simulink model "TST_AccPed_DrvDemDes"  (R2016b)
settings: Solver=FixedStepDiscrete  StartTime=0.0  StopTime=simTime  FixedStep=sampleTime  RelTol=1e-3
values from neighbouring files (symbols this model uses):
  testCase = 1    [initTST_AccPed_DrvDemDes_001.m]    (also in initTST_AccPed_DrvDemDes_002.m = 2; initTST_AccPed_DrvDemDes_003.m = 3; initTST_AccPed_DrvDemDes_004.m = 4; initTST_AccPed_DrvDemDes_005.m = 5)
libraries: simulink x61, UnitTest_Lib x54
(part 2 of 2)

== system TST_AccPed_DrvDemDes/simulationInput/testSignals_R001 ==
  BC : BusCreator  Inputs=22
  spec_APP_r : FromWorkspace  VariableName=testSig_APP_r  Interpolate=off  OutputAfterFinalValue=Holding final value
  spec_AccPed_facCompAcs : FromWorkspace  VariableName=testSig_AccPed_facCompAcs  Interpolate=off  OutputAfterFinalValue=Holding final value
  spec_AccPed_rBrk50_mp : FromWorkspace  VariableName=testSig_AccPed_rBrk50_mp  Interpolate=off  OutputAfterFinalValue=Holding final value
  spec_AccPed_rTrq : FromWorkspace  VariableName=testSig_AccPed_rTrq  Interpolate=off  OutputAfterFinalValue=Holding final value
  spec_AccPed_stBrkDes : FromWorkspace  VariableName=testSig_AccPed_stBrkDes  Interpolate=off  OutputAfterFinalValue=Holding final value
  spec_AccPed_stBrkDes_mp : FromWorkspace  VariableName=testSig_AccPed_stBrkDes_mp  Interpolate=off  OutputAfterFinalValue=Holding final value
  spec_AccPed_stMS : FromWorkspace  VariableName=testSig_AccPed_stMS  Interpolate=off  OutputAfterFinalValue=Holding final value
  spec_AccPed_trqComp : FromWorkspace  VariableName=testSig_AccPed_trqComp  Interpolate=off  OutputAfterFinalValue=Holding final value
  spec_AccPed_trqDesAct : FromWorkspace  VariableName=testSig_AccPed_trqDesAct  Interpolate=off  OutputAfterFinalValue=Holding final value
  spec_AccPed_trqDesPull : FromWorkspace  VariableName=testSig_AccPed_trqDesPull  Interpolate=off  OutputAfterFinalValue=Holding final value
  spec_AccPed_trqDifBrk_mp : FromWorkspace  VariableName=testSig_AccPed_trqDifBrk_mp  Interpolate=off  OutputAfterFinalValue=Holding final value
  spec_AccPed_trqLimMax : FromWorkspace  VariableName=testSig_AccPed_trqLimMax  Interpolate=off  OutputAfterFinalValue=Holding final value
  spec_Brk_st : FromWorkspace  VariableName=testSig_Brk_st  Interpolate=off  OutputAfterFinalValue=Holding final value
  spec_CoME_trqDesComp : FromWorkspace  VariableName=testSig_CoME_trqDesComp  Interpolate=off  OutputAfterFinalValue=Holding final value
  spec_DrvDem_swtDrvNGovActv : FromWorkspace  VariableName=testSig_DrvDem_swtDrvNGovActv  Interpolate=off  OutputAfterFinalValue=Holding final value
  spec_EBrk_st : FromWorkspace  VariableName=testSig_EBrk_st  Interpolate=off  OutputAfterFinalValue=Holding final value
  spec_Epm_nEng : FromWorkspace  VariableName=testSig_Epm_nEng  Interpolate=off  OutputAfterFinalValue=Holding final value
  spec_GlbDa_vX : FromWorkspace  VariableName=testSig_GlbDa_vX  Interpolate=off  OutputAfterFinalValue=Holding final value
  spec_PT_stTraRevGear : FromWorkspace  VariableName=testSig_PT_stTraRevGear  Interpolate=off  OutputAfterFinalValue=Holding final value
  spec_PT_trqWhlMinEng : FromWorkspace  VariableName=testSig_PT_trqWhlMinEng  Interpolate=off  OutputAfterFinalValue=Holding final value
  spec_PT_trqWhlMinEngBrk : FromWorkspace  VariableName=testSig_PT_trqWhlMinEngBrk  Interpolate=off  OutputAfterFinalValue=Holding final value
  spec_VehMot_stPrpAccPed : FromWorkspace  VariableName=testSig_VehMot_stPrpAccPed  Interpolate=off  OutputAfterFinalValue=Holding final value
  testSignals : Outport
  wires:
  BC/1 -> testSignals/1
  spec_PT_trqWhlMinEng/1 -> BC/1  "testSig_PT_trqWhlMinEng"
  spec_APP_r/1 -> BC/2  "testSig_APP_r"
  spec_Epm_nEng/1 -> BC/3  "testSig_Epm_nEng"
  spec_GlbDa_vX/1 -> BC/4  "testSig_GlbDa_vX"
  spec_CoME_trqDesComp/1 -> BC/5  "testSig_CoME_trqDesComp"
  spec_DrvDem_swtDrvNGovActv/1 -> BC/6  "testSig_DrvDem_swtDrvNGovActv"
  spec_Brk_st/1 -> BC/7  "testSig_Brk_st"
  spec_EBrk_st/1 -> BC/8  "testSig_EBrk_st"
  spec_PT_trqWhlMinEngBrk/1 -> BC/9  "testSig_PT_trqWhlMinEngBrk"
  spec_AccPed_trqLimMax/1 -> BC/10  "testSig_AccPed_trqLimMax"
  spec_AccPed_rTrq/1 -> BC/11  "testSig_AccPed_rTrq"
  spec_AccPed_stMS/1 -> BC/12  "testSig_AccPed_stMS"
  spec_PT_stTraRevGear/1 -> BC/13  "testSig_PT_stTraRevGear"
  spec_AccPed_trqDesAct/1 -> BC/14  "testSig_AccPed_trqDesAct"
  spec_VehMot_stPrpAccPed/1 -> BC/15  "testSig_VehMot_stPrpAccPed"
  spec_AccPed_facCompAcs/1 -> BC/16  "testSig_AccPed_facCompAcs"
  spec_AccPed_trqComp/1 -> BC/17  "testSig_AccPed_trqComp"
  spec_AccPed_stBrkDes/1 -> BC/18  "testSig_AccPed_stBrkDes"
  spec_AccPed_stBrkDes_mp/1 -> BC/19  "testSig_AccPed_stBrkDes_mp"
  spec_AccPed_trqDifBrk_mp/1 -> BC/20  "testSig_AccPed_trqDifBrk_mp"
  spec_AccPed_rBrk50_mp/1 -> BC/21  "testSig_AccPed_rBrk50_mp"
  spec_AccPed_trqDesPull/1 -> BC/22  "testSig_AccPed_trqDesPull"

== system TST_AccPed_DrvDemDes/simulationInput/testSignals_R002 ==
  BC : BusCreator  Inputs=22
  spec_APP_r : FromWorkspace  VariableName=testSig_APP_r  Interpolate=off  OutputAfterFinalValue=Holding final value
  spec_AccPed_facCompAcs : FromWorkspace  VariableName=testSig_AccPed_facCompAcs  Interpolate=off  OutputAfterFinalValue=Holding final value
  spec_AccPed_rBrk50_mp : FromWorkspace  VariableName=testSig_AccPed_rBrk50_mp  Interpolate=off  OutputAfterFinalValue=Holding final value
  spec_AccPed_rTrq : FromWorkspace  VariableName=testSig_AccPed_rTrq  Interpolate=off  OutputAfterFinalValue=Holding final value
  spec_AccPed_stBrkDes : FromWorkspace  VariableName=testSig_AccPed_stBrkDes  Interpolate=off  OutputAfterFinalValue=Holding final value
  spec_AccPed_stBrkDes_mp : FromWorkspace  VariableName=testSig_AccPed_stBrkDes_mp  Interpolate=off  OutputAfterFinalValue=Holding final value
  spec_AccPed_stMS : FromWorkspace  VariableName=testSig_AccPed_stMS  Interpolate=off  OutputAfterFinalValue=Holding final value
  spec_AccPed_trqComp : FromWorkspace  VariableName=testSig_AccPed_trqComp  Interpolate=off  OutputAfterFinalValue=Holding final value
  spec_AccPed_trqDesAct : FromWorkspace  VariableName=testSig_AccPed_trqDesAct  Interpolate=off  OutputAfterFinalValue=Holding final value
  spec_AccPed_trqDesPull : FromWorkspace  VariableName=testSig_AccPed_trqDesPull  Interpolate=off  OutputAfterFinalValue=Holding final value
  spec_AccPed_trqDifBrk_mp : FromWorkspace  VariableName=testSig_AccPed_trqDifBrk_mp  Interpolate=off  OutputAfterFinalValue=Holding final value
  spec_AccPed_trqLimMax : FromWorkspace  VariableName=testSig_AccPed_trqLimMax  Interpolate=off  OutputAfterFinalValue=Holding final value
  spec_Brk_st : FromWorkspace  VariableName=testSig_Brk_st  Interpolate=off  OutputAfterFinalValue=Holding final value
  spec_CoME_trqDesComp : FromWorkspace  VariableName=testSig_CoME_trqDesComp  Interpolate=off  OutputAfterFinalValue=Holding final value
  spec_DrvDem_swtDrvNGovActv : FromWorkspace  VariableName=testSig_DrvDem_swtDrvNGovActv  Interpolate=off  OutputAfterFinalValue=Holding final value
  spec_EBrk_st : FromWorkspace  VariableName=testSig_EBrk_st  Interpolate=off  OutputAfterFinalValue=Holding final value
  spec_Epm_nEng : FromWorkspace  VariableName=testSig_Epm_nEng  Interpolate=off  OutputAfterFinalValue=Holding final value
  spec_GlbDa_vX : FromWorkspace  VariableName=testSig_GlbDa_vX  Interpolate=off  OutputAfterFinalValue=Holding final value
  spec_PT_stTraRevGear : FromWorkspace  VariableName=testSig_PT_stTraRevGear  Interpolate=off  OutputAfterFinalValue=Holding final value
  spec_PT_trqWhlMinEng : FromWorkspace  VariableName=testSig_PT_trqWhlMinEng  Interpolate=off  OutputAfterFinalValue=Holding final value
  spec_PT_trqWhlMinEngBrk : FromWorkspace  VariableName=testSig_PT_trqWhlMinEngBrk  Interpolate=off  OutputAfterFinalValue=Holding final value
  spec_VehMot_stPrpAccPed : FromWorkspace  VariableName=testSig_VehMot_stPrpAccPed  Interpolate=off  OutputAfterFinalValue=Holding final value
  testSignals : Outport
  wires:
  BC/1 -> testSignals/1
  spec_PT_trqWhlMinEng/1 -> BC/1  "testSig_PT_trqWhlMinEng"
  spec_APP_r/1 -> BC/2  "testSig_APP_r"
  spec_Epm_nEng/1 -> BC/3  "testSig_Epm_nEng"
  spec_GlbDa_vX/1 -> BC/4  "testSig_GlbDa_vX"
  spec_CoME_trqDesComp/1 -> BC/5  "testSig_CoME_trqDesComp"
  spec_DrvDem_swtDrvNGovActv/1 -> BC/6  "testSig_DrvDem_swtDrvNGovActv"
  spec_Brk_st/1 -> BC/7  "testSig_Brk_st"
  spec_EBrk_st/1 -> BC/8  "testSig_EBrk_st"
  spec_PT_trqWhlMinEngBrk/1 -> BC/9  "testSig_PT_trqWhlMinEngBrk"
  spec_AccPed_trqLimMax/1 -> BC/10  "testSig_AccPed_trqLimMax"
  spec_AccPed_rTrq/1 -> BC/11  "testSig_AccPed_rTrq"
  spec_AccPed_stMS/1 -> BC/12  "testSig_AccPed_stMS"
  spec_PT_stTraRevGear/1 -> BC/13  "testSig_PT_stTraRevGear"
  spec_AccPed_trqDesAct/1 -> BC/14  "testSig_AccPed_trqDesAct"
  spec_VehMot_stPrpAccPed/1 -> BC/15  "testSig_VehMot_stPrpAccPed"
  spec_AccPed_facCompAcs/1 -> BC/16  "testSig_AccPed_facCompAcs"
  spec_AccPed_trqComp/1 -> BC/17  "testSig_AccPed_trqComp"
  spec_AccPed_stBrkDes/1 -> BC/18  "testSig_AccPed_stBrkDes"
  spec_AccPed_stBrkDes_mp/1 -> BC/19  "testSig_AccPed_stBrkDes_mp"
  spec_AccPed_trqDifBrk_mp/1 -> BC/20  "testSig_AccPed_trqDifBrk_mp"
  spec_AccPed_rBrk50_mp/1 -> BC/21  "testSig_AccPed_rBrk50_mp"
  spec_AccPed_trqDesPull/1 -> BC/22  "testSig_AccPed_trqDesPull"

== system TST_AccPed_DrvDemDes/simulationInput/testSignals_R003 ==
  BC : BusCreator  Inputs=22
  spec_APP_r : FromWorkspace  VariableName=testSig_APP_r  Interpolate=off  OutputAfterFinalValue=Holding final value
  spec_AccPed_facCompAcs : FromWorkspace  VariableName=testSig_AccPed_facCompAcs  Interpolate=off  OutputAfterFinalValue=Holding final value
  spec_AccPed_rBrk50_mp : FromWorkspace  VariableName=testSig_AccPed_rBrk50_mp  Interpolate=off  OutputAfterFinalValue=Holding final value
  spec_AccPed_rTrq : FromWorkspace  VariableName=testSig_AccPed_rTrq  Interpolate=off  OutputAfterFinalValue=Holding final value
  spec_AccPed_stBrkDes : FromWorkspace  VariableName=testSig_AccPed_stBrkDes  Interpolate=off  OutputAfterFinalValue=Holding final value
  spec_AccPed_stBrkDes_mp : FromWorkspace  VariableName=testSig_AccPed_stBrkDes_mp  Interpolate=off  OutputAfterFinalValue=Holding final value
  spec_AccPed_stMS : FromWorkspace  VariableName=testSig_AccPed_stMS  Interpolate=off  OutputAfterFinalValue=Holding final value
  spec_AccPed_trqComp : FromWorkspace  VariableName=testSig_AccPed_trqComp  Interpolate=off  OutputAfterFinalValue=Holding final value
  spec_AccPed_trqDesAct : FromWorkspace  VariableName=testSig_AccPed_trqDesAct  Interpolate=off  OutputAfterFinalValue=Holding final value
  spec_AccPed_trqDesPull : FromWorkspace  VariableName=testSig_AccPed_trqDesPull  Interpolate=off  OutputAfterFinalValue=Holding final value
  spec_AccPed_trqDifBrk_mp : FromWorkspace  VariableName=testSig_AccPed_trqDifBrk_mp  Interpolate=off  OutputAfterFinalValue=Holding final value
  spec_AccPed_trqLimMax : FromWorkspace  VariableName=testSig_AccPed_trqLimMax  Interpolate=off  OutputAfterFinalValue=Holding final value
  spec_Brk_st : FromWorkspace  VariableName=testSig_Brk_st  Interpolate=off  OutputAfterFinalValue=Holding final value
  spec_CoME_trqDesComp : FromWorkspace  VariableName=testSig_CoME_trqDesComp  Interpolate=off  OutputAfterFinalValue=Holding final value
  spec_DrvDem_swtDrvNGovActv : FromWorkspace  VariableName=testSig_DrvDem_swtDrvNGovActv  Interpolate=off  OutputAfterFinalValue=Holding final value
  spec_EBrk_st : FromWorkspace  VariableName=testSig_EBrk_st  Interpolate=off  OutputAfterFinalValue=Holding final value
  spec_Epm_nEng : FromWorkspace  VariableName=testSig_Epm_nEng  Interpolate=off  OutputAfterFinalValue=Holding final value
  spec_GlbDa_vX : FromWorkspace  VariableName=testSig_GlbDa_vX  Interpolate=off  OutputAfterFinalValue=Holding final value
  spec_PT_stTraRevGear : FromWorkspace  VariableName=testSig_PT_stTraRevGear  Interpolate=off  OutputAfterFinalValue=Holding final value
  spec_PT_trqWhlMinEng : FromWorkspace  VariableName=testSig_PT_trqWhlMinEng  Interpolate=off  OutputAfterFinalValue=Holding final value
  spec_PT_trqWhlMinEngBrk : FromWorkspace  VariableName=testSig_PT_trqWhlMinEngBrk  Interpolate=off  OutputAfterFinalValue=Holding final value
  spec_VehMot_stPrpAccPed : FromWorkspace  VariableName=testSig_VehMot_stPrpAccPed  Interpolate=off  OutputAfterFinalValue=Holding final value
  testSignals : Outport
  wires:
  BC/1 -> testSignals/1
  spec_PT_trqWhlMinEng/1 -> BC/1  "testSig_PT_trqWhlMinEng"
  spec_APP_r/1 -> BC/2  "testSig_APP_r"
  spec_Epm_nEng/1 -> BC/3  "testSig_Epm_nEng"
  spec_GlbDa_vX/1 -> BC/4  "testSig_GlbDa_vX"
  spec_CoME_trqDesComp/1 -> BC/5  "testSig_CoME_trqDesComp"
  spec_DrvDem_swtDrvNGovActv/1 -> BC/6  "testSig_DrvDem_swtDrvNGovActv"
  spec_Brk_st/1 -> BC/7  "testSig_Brk_st"
  spec_EBrk_st/1 -> BC/8  "testSig_EBrk_st"
  spec_PT_trqWhlMinEngBrk/1 -> BC/9  "testSig_PT_trqWhlMinEngBrk"
  spec_AccPed_trqLimMax/1 -> BC/10  "testSig_AccPed_trqLimMax"
  spec_AccPed_rTrq/1 -> BC/11  "testSig_AccPed_rTrq"
  spec_AccPed_stMS/1 -> BC/12  "testSig_AccPed_stMS"
  spec_PT_stTraRevGear/1 -> BC/13  "testSig_PT_stTraRevGear"
  spec_AccPed_trqDesAct/1 -> BC/14  "testSig_AccPed_trqDesAct"
  spec_VehMot_stPrpAccPed/1 -> BC/15  "testSig_VehMot_stPrpAccPed"
  spec_AccPed_facCompAcs/1 -> BC/16  "testSig_AccPed_facCompAcs"
  spec_AccPed_trqComp/1 -> BC/17  "testSig_AccPed_trqComp"
  spec_AccPed_stBrkDes/1 -> BC/18  "testSig_AccPed_stBrkDes"
  spec_AccPed_stBrkDes_mp/1 -> BC/19  "testSig_AccPed_stBrkDes_mp"
  spec_AccPed_trqDifBrk_mp/1 -> BC/20  "testSig_AccPed_trqDifBrk_mp"
  spec_AccPed_rBrk50_mp/1 -> BC/21  "testSig_AccPed_rBrk50_mp"
  spec_AccPed_trqDesPull/1 -> BC/22  "testSig_AccPed_trqDesPull"

== system TST_AccPed_DrvDemDes/simulationInput/testSignals_R004 ==
  BC : BusCreator  Inputs=22
  spec_APP_r : FromWorkspace  VariableName=testSig_APP_r  Interpolate=off  OutputAfterFinalValue=Holding final value
  spec_AccPed_facCompAcs : FromWorkspace  VariableName=testSig_AccPed_facCompAcs  Interpolate=off  OutputAfterFinalValue=Holding final value
  spec_AccPed_rBrk50_mp : FromWorkspace  VariableName=testSig_AccPed_rBrk50_mp  Interpolate=off  OutputAfterFinalValue=Holding final value
  spec_AccPed_rTrq : FromWorkspace  VariableName=testSig_AccPed_rTrq  Interpolate=off  OutputAfterFinalValue=Holding final value
  spec_AccPed_stBrkDes : FromWorkspace  VariableName=testSig_AccPed_stBrkDes  Interpolate=off  OutputAfterFinalValue=Holding final value
  spec_AccPed_stBrkDes_mp : FromWorkspace  VariableName=testSig_AccPed_stBrkDes_mp  Interpolate=off  OutputAfterFinalValue=Holding final value
  spec_AccPed_stMS : FromWorkspace  VariableName=testSig_AccPed_stMS  Interpolate=off  OutputAfterFinalValue=Holding final value
  spec_AccPed_trqComp : FromWorkspace  VariableName=testSig_AccPed_trqComp  Interpolate=off  OutputAfterFinalValue=Holding final value
  spec_AccPed_trqDesAct : FromWorkspace  VariableName=testSig_AccPed_trqDesAct  Interpolate=off  OutputAfterFinalValue=Holding final value
  spec_AccPed_trqDesPull : FromWorkspace  VariableName=testSig_AccPed_trqDesPull  Interpolate=off  OutputAfterFinalValue=Holding final value
  spec_AccPed_trqDifBrk_mp : FromWorkspace  VariableName=testSig_AccPed_trqDifBrk_mp  Interpolate=off  OutputAfterFinalValue=Holding final value
  spec_AccPed_trqLimMax : FromWorkspace  VariableName=testSig_AccPed_trqLimMax  Interpolate=off  OutputAfterFinalValue=Holding final value
  spec_Brk_st : FromWorkspace  VariableName=testSig_Brk_st  Interpolate=off  OutputAfterFinalValue=Holding final value
  spec_CoME_trqDesComp : FromWorkspace  VariableName=testSig_CoME_trqDesComp  Interpolate=off  OutputAfterFinalValue=Holding final value
  spec_DrvDem_swtDrvNGovActv : FromWorkspace  VariableName=testSig_DrvDem_swtDrvNGovActv  Interpolate=off  OutputAfterFinalValue=Holding final value
  spec_EBrk_st : FromWorkspace  VariableName=testSig_EBrk_st  Interpolate=off  OutputAfterFinalValue=Holding final value
  spec_Epm_nEng : FromWorkspace  VariableName=testSig_Epm_nEng  Interpolate=off  OutputAfterFinalValue=Holding final value
  spec_GlbDa_vX : FromWorkspace  VariableName=testSig_GlbDa_vX  Interpolate=off  OutputAfterFinalValue=Holding final value
  spec_PT_stTraRevGear : FromWorkspace  VariableName=testSig_PT_stTraRevGear  Interpolate=off  OutputAfterFinalValue=Holding final value
  spec_PT_trqWhlMinEng : FromWorkspace  VariableName=testSig_PT_trqWhlMinEng  Interpolate=off  OutputAfterFinalValue=Holding final value
  spec_PT_trqWhlMinEngBrk : FromWorkspace  VariableName=testSig_PT_trqWhlMinEngBrk  Interpolate=off  OutputAfterFinalValue=Holding final value
  spec_VehMot_stPrpAccPed : FromWorkspace  VariableName=testSig_VehMot_stPrpAccPed  Interpolate=off  OutputAfterFinalValue=Holding final value
  testSignals : Outport
  wires:
  BC/1 -> testSignals/1
  spec_PT_trqWhlMinEng/1 -> BC/1  "testSig_PT_trqWhlMinEng"
  spec_APP_r/1 -> BC/2  "testSig_APP_r"
  spec_Epm_nEng/1 -> BC/3  "testSig_Epm_nEng"
  spec_GlbDa_vX/1 -> BC/4  "testSig_GlbDa_vX"
  spec_CoME_trqDesComp/1 -> BC/5  "testSig_CoME_trqDesComp"
  spec_DrvDem_swtDrvNGovActv/1 -> BC/6  "testSig_DrvDem_swtDrvNGovActv"
  spec_Brk_st/1 -> BC/7  "testSig_Brk_st"
  spec_EBrk_st/1 -> BC/8  "testSig_EBrk_st"
  spec_PT_trqWhlMinEngBrk/1 -> BC/9  "testSig_PT_trqWhlMinEngBrk"
  spec_AccPed_trqLimMax/1 -> BC/10  "testSig_AccPed_trqLimMax"
  spec_AccPed_rTrq/1 -> BC/11  "testSig_AccPed_rTrq"
  spec_AccPed_stMS/1 -> BC/12  "testSig_AccPed_stMS"
  spec_PT_stTraRevGear/1 -> BC/13  "testSig_PT_stTraRevGear"
  spec_AccPed_trqDesAct/1 -> BC/14  "testSig_AccPed_trqDesAct"
  spec_VehMot_stPrpAccPed/1 -> BC/15  "testSig_VehMot_stPrpAccPed"
  spec_AccPed_facCompAcs/1 -> BC/16  "testSig_AccPed_facCompAcs"
  spec_AccPed_trqComp/1 -> BC/17  "testSig_AccPed_trqComp"
  spec_AccPed_stBrkDes/1 -> BC/18  "testSig_AccPed_stBrkDes"
  spec_AccPed_stBrkDes_mp/1 -> BC/19  "testSig_AccPed_stBrkDes_mp"
  spec_AccPed_trqDifBrk_mp/1 -> BC/20  "testSig_AccPed_trqDifBrk_mp"
  spec_AccPed_rBrk50_mp/1 -> BC/21  "testSig_AccPed_rBrk50_mp"
  spec_AccPed_trqDesPull/1 -> BC/22  "testSig_AccPed_trqDesPull"

== system TST_AccPed_DrvDemDes/simulationInput/testSignals_R005 ==
  BC : BusCreator  Inputs=22
  spec_APP_r : FromWorkspace  VariableName=testSig_APP_r  Interpolate=off  OutputAfterFinalValue=Holding final value
  spec_AccPed_facCompAcs : FromWorkspace  VariableName=testSig_AccPed_facCompAcs  Interpolate=off  OutputAfterFinalValue=Holding final value
  spec_AccPed_rBrk50_mp : FromWorkspace  VariableName=testSig_AccPed_rBrk50_mp  Interpolate=off  OutputAfterFinalValue=Holding final value
  spec_AccPed_rTrq : FromWorkspace  VariableName=testSig_AccPed_rTrq  Interpolate=off  OutputAfterFinalValue=Holding final value
  spec_AccPed_stBrkDes : FromWorkspace  VariableName=testSig_AccPed_stBrkDes  Interpolate=off  OutputAfterFinalValue=Holding final value
  spec_AccPed_stBrkDes_mp : FromWorkspace  VariableName=testSig_AccPed_stBrkDes_mp  Interpolate=off  OutputAfterFinalValue=Holding final value
  spec_AccPed_stMS : FromWorkspace  VariableName=testSig_AccPed_stMS  Interpolate=off  OutputAfterFinalValue=Holding final value
  spec_AccPed_trqComp : FromWorkspace  VariableName=testSig_AccPed_trqComp  Interpolate=off  OutputAfterFinalValue=Holding final value
  spec_AccPed_trqDesAct : FromWorkspace  VariableName=testSig_AccPed_trqDesAct  Interpolate=off  OutputAfterFinalValue=Holding final value
  spec_AccPed_trqDesPull : FromWorkspace  VariableName=testSig_AccPed_trqDesPull  Interpolate=off  OutputAfterFinalValue=Holding final value
  spec_AccPed_trqDifBrk_mp : FromWorkspace  VariableName=testSig_AccPed_trqDifBrk_mp  Interpolate=off  OutputAfterFinalValue=Holding final value
  spec_AccPed_trqLimMax : FromWorkspace  VariableName=testSig_AccPed_trqLimMax  Interpolate=off  OutputAfterFinalValue=Holding final value
  spec_Brk_st : FromWorkspace  VariableName=testSig_Brk_st  Interpolate=off  OutputAfterFinalValue=Holding final value
  spec_CoME_trqDesComp : FromWorkspace  VariableName=testSig_CoME_trqDesComp  Interpolate=off  OutputAfterFinalValue=Holding final value
  spec_DrvDem_swtDrvNGovActv : FromWorkspace  VariableName=testSig_DrvDem_swtDrvNGovActv  Interpolate=off  OutputAfterFinalValue=Holding final value
  spec_EBrk_st : FromWorkspace  VariableName=testSig_EBrk_st  Interpolate=off  OutputAfterFinalValue=Holding final value
  spec_Epm_nEng : FromWorkspace  VariableName=testSig_Epm_nEng  Interpolate=off  OutputAfterFinalValue=Holding final value
  spec_GlbDa_vX : FromWorkspace  VariableName=testSig_GlbDa_vX  Interpolate=off  OutputAfterFinalValue=Holding final value
  spec_PT_stTraRevGear : FromWorkspace  VariableName=testSig_PT_stTraRevGear  Interpolate=off  OutputAfterFinalValue=Holding final value
  spec_PT_trqWhlMinEng : FromWorkspace  VariableName=testSig_PT_trqWhlMinEng  Interpolate=off  OutputAfterFinalValue=Holding final value
  spec_PT_trqWhlMinEngBrk : FromWorkspace  VariableName=testSig_PT_trqWhlMinEngBrk  Interpolate=off  OutputAfterFinalValue=Holding final value
  spec_VehMot_stPrpAccPed : FromWorkspace  VariableName=testSig_VehMot_stPrpAccPed  Interpolate=off  OutputAfterFinalValue=Holding final value
  testSignals : Outport
  wires:
  BC/1 -> testSignals/1
  spec_PT_trqWhlMinEng/1 -> BC/1  "testSig_PT_trqWhlMinEng"
  spec_APP_r/1 -> BC/2  "testSig_APP_r"
  spec_Epm_nEng/1 -> BC/3  "testSig_Epm_nEng"
  spec_GlbDa_vX/1 -> BC/4  "testSig_GlbDa_vX"
  spec_CoME_trqDesComp/1 -> BC/5  "testSig_CoME_trqDesComp"
  spec_DrvDem_swtDrvNGovActv/1 -> BC/6  "testSig_DrvDem_swtDrvNGovActv"
  spec_Brk_st/1 -> BC/7  "testSig_Brk_st"
  spec_EBrk_st/1 -> BC/8  "testSig_EBrk_st"
  spec_PT_trqWhlMinEngBrk/1 -> BC/9  "testSig_PT_trqWhlMinEngBrk"
  spec_AccPed_trqLimMax/1 -> BC/10  "testSig_AccPed_trqLimMax"
  spec_AccPed_rTrq/1 -> BC/11  "testSig_AccPed_rTrq"
  spec_AccPed_stMS/1 -> BC/12  "testSig_AccPed_stMS"
  spec_PT_stTraRevGear/1 -> BC/13  "testSig_PT_stTraRevGear"
  spec_AccPed_trqDesAct/1 -> BC/14  "testSig_AccPed_trqDesAct"
  spec_VehMot_stPrpAccPed/1 -> BC/15  "testSig_VehMot_stPrpAccPed"
  spec_AccPed_facCompAcs/1 -> BC/16  "testSig_AccPed_facCompAcs"
  spec_AccPed_trqComp/1 -> BC/17  "testSig_AccPed_trqComp"
  spec_AccPed_stBrkDes/1 -> BC/18  "testSig_AccPed_stBrkDes"
  spec_AccPed_stBrkDes_mp/1 -> BC/19  "testSig_AccPed_stBrkDes_mp"
  spec_AccPed_trqDifBrk_mp/1 -> BC/20  "testSig_AccPed_trqDifBrk_mp"
  spec_AccPed_rBrk50_mp/1 -> BC/21  "testSig_AccPed_rBrk50_mp"
  spec_AccPed_trqDesPull/1 -> BC/22  "testSig_AccPed_trqDesPull"

== system TST_AccPed_DrvDemDes/simulationInput/testSignals_R006 ==
  BC : BusCreator  Inputs=22
  spec_APP_r : FromWorkspace  VariableName=testSig_APP_r  Interpolate=off  OutputAfterFinalValue=Holding final value
  spec_AccPed_facCompAcs : FromWorkspace  VariableName=testSig_AccPed_facCompAcs  Interpolate=off  OutputAfterFinalValue=Holding final value
  spec_AccPed_rBrk50_mp : FromWorkspace  VariableName=testSig_AccPed_rBrk50_mp  Interpolate=off  OutputAfterFinalValue=Holding final value
  spec_AccPed_rTrq : FromWorkspace  VariableName=testSig_AccPed_rTrq  Interpolate=off  OutputAfterFinalValue=Holding final value
  spec_AccPed_stBrkDes : FromWorkspace  VariableName=testSig_AccPed_stBrkDes  Interpolate=off  OutputAfterFinalValue=Holding final value
  spec_AccPed_stBrkDes_mp : FromWorkspace  VariableName=testSig_AccPed_stBrkDes_mp  Interpolate=off  OutputAfterFinalValue=Holding final value
  spec_AccPed_stMS : FromWorkspace  VariableName=testSig_AccPed_stMS  Interpolate=off  OutputAfterFinalValue=Holding final value
  spec_AccPed_trqComp : FromWorkspace  VariableName=testSig_AccPed_trqComp  Interpolate=off  OutputAfterFinalValue=Holding final value
  spec_AccPed_trqDesAct : FromWorkspace  VariableName=testSig_AccPed_trqDesAct  Interpolate=off  OutputAfterFinalValue=Holding final value
  spec_AccPed_trqDesPull : FromWorkspace  VariableName=testSig_AccPed_trqDesPull  Interpolate=off  OutputAfterFinalValue=Holding final value
  spec_AccPed_trqDifBrk_mp : FromWorkspace  VariableName=testSig_AccPed_trqDifBrk_mp  Interpolate=off  OutputAfterFinalValue=Holding final value
  spec_AccPed_trqLimMax : FromWorkspace  VariableName=testSig_AccPed_trqLimMax  Interpolate=off  OutputAfterFinalValue=Holding final value
  spec_Brk_st : FromWorkspace  VariableName=testSig_Brk_st  Interpolate=off  OutputAfterFinalValue=Holding final value
  spec_CoME_trqDesComp : FromWorkspace  VariableName=testSig_CoME_trqDesComp  Interpolate=off  OutputAfterFinalValue=Holding final value
  spec_DrvDem_swtDrvNGovActv : FromWorkspace  VariableName=testSig_DrvDem_swtDrvNGovActv  Interpolate=off  OutputAfterFinalValue=Holding final value
  spec_EBrk_st : FromWorkspace  VariableName=testSig_EBrk_st  Interpolate=off  OutputAfterFinalValue=Holding final value
  spec_Epm_nEng : FromWorkspace  VariableName=testSig_Epm_nEng  Interpolate=off  OutputAfterFinalValue=Holding final value
  spec_GlbDa_vX : FromWorkspace  VariableName=testSig_GlbDa_vX  Interpolate=off  OutputAfterFinalValue=Holding final value
  spec_PT_stTraRevGear : FromWorkspace  VariableName=testSig_PT_stTraRevGear  Interpolate=off  OutputAfterFinalValue=Holding final value
  spec_PT_trqWhlMinEng : FromWorkspace  VariableName=testSig_PT_trqWhlMinEng  Interpolate=off  OutputAfterFinalValue=Holding final value
  spec_PT_trqWhlMinEngBrk : FromWorkspace  VariableName=testSig_PT_trqWhlMinEngBrk  Interpolate=off  OutputAfterFinalValue=Holding final value
  spec_VehMot_stPrpAccPed : FromWorkspace  VariableName=testSig_VehMot_stPrpAccPed  Interpolate=off  OutputAfterFinalValue=Holding final value
  testSignals : Outport
  wires:
  BC/1 -> testSignals/1
  spec_PT_trqWhlMinEng/1 -> BC/1  "testSig_PT_trqWhlMinEng"
  spec_APP_r/1 -> BC/2  "testSig_APP_r"
  spec_Epm_nEng/1 -> BC/3  "testSig_Epm_nEng"
  spec_GlbDa_vX/1 -> BC/4  "testSig_GlbDa_vX"
  spec_CoME_trqDesComp/1 -> BC/5  "testSig_CoME_trqDesComp"
  spec_DrvDem_swtDrvNGovActv/1 -> BC/6  "testSig_DrvDem_swtDrvNGovActv"
  spec_Brk_st/1 -> BC/7  "testSig_Brk_st"
  spec_EBrk_st/1 -> BC/8  "testSig_EBrk_st"
  spec_PT_trqWhlMinEngBrk/1 -> BC/9  "testSig_PT_trqWhlMinEngBrk"
  spec_AccPed_trqLimMax/1 -> BC/10  "testSig_AccPed_trqLimMax"
  spec_AccPed_rTrq/1 -> BC/11  "testSig_AccPed_rTrq"
  spec_AccPed_stMS/1 -> BC/12  "testSig_AccPed_stMS"
  spec_PT_stTraRevGear/1 -> BC/13  "testSig_PT_stTraRevGear"
  spec_AccPed_trqDesAct/1 -> BC/14  "testSig_AccPed_trqDesAct"
  spec_VehMot_stPrpAccPed/1 -> BC/15  "testSig_VehMot_stPrpAccPed"
  spec_AccPed_facCompAcs/1 -> BC/16  "testSig_AccPed_facCompAcs"
  spec_AccPed_trqComp/1 -> BC/17  "testSig_AccPed_trqComp"
  spec_AccPed_stBrkDes/1 -> BC/18  "testSig_AccPed_stBrkDes"
  spec_AccPed_stBrkDes_mp/1 -> BC/19  "testSig_AccPed_stBrkDes_mp"
  spec_AccPed_trqDifBrk_mp/1 -> BC/20  "testSig_AccPed_trqDifBrk_mp"
  spec_AccPed_rBrk50_mp/1 -> BC/21  "testSig_AccPed_rBrk50_mp"
  spec_AccPed_trqDesPull/1 -> BC/22  "testSig_AccPed_trqDesPull"

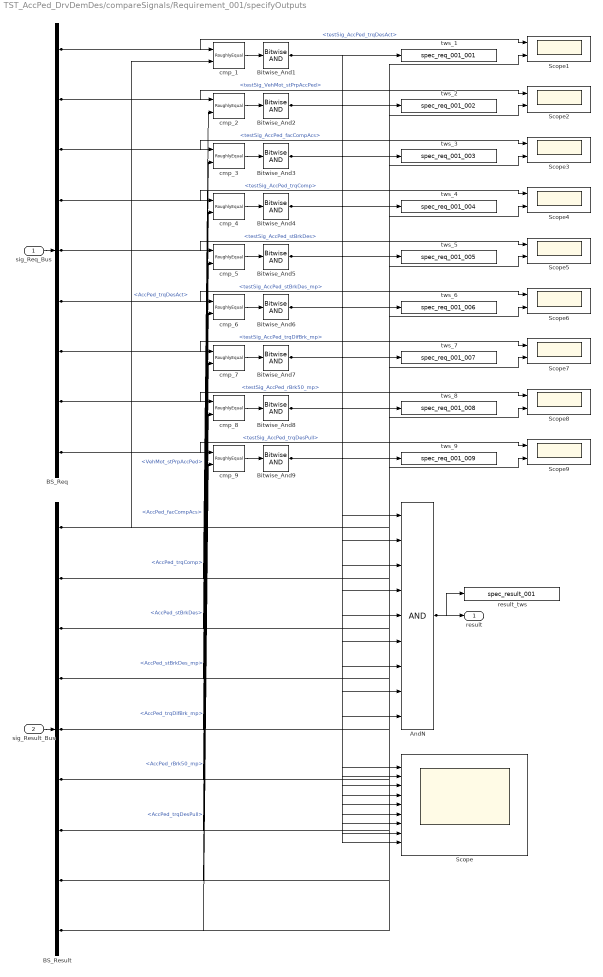
== system TST_AccPed_DrvDemDes/compareSignals/Requirement_001/specifyOutputs ==
  sig_Req_Bus : Inport
  sig_Result_Bus : Inport  Port=2
  AndN : Logic  Inputs=9
  BS_Req : BusSelector  OutputSignals=testSig_AccPed_trqDesAct,testSig_VehMot_stPrpAccPed,testSig_AccPed_facCompAcs,testSig_AccPed_trqComp,testSig_AccPed_stBrkDes,testSig_AccPed_stBrkDes_mp,testSig_AccPed_trqDifBrk_mp,testSig_AccPed_rBrk50_mp,testSig_AccPed_trqDesPull
  BS_Result : BusSelector  OutputSignals=AccPed_trqDesAct,VehMot_stPrpAccPed,AccPed_facCompAcs,AccPed_trqComp,AccPed_stBrkDes,AccPed_stBrkDes_mp,AccPed_trqDifBrk_mp,AccPed_rBrk50_mp,AccPed_trqDesPull
  Bitwise_And{1..9} (9 alike) : simulink/Logic and Bit Operations/Bitwise Operator  logicop=AND  UseBitMask=off  BitMask=bin2dec('11011001')  BitMaskRealWorld=Stored Integer
  Scope : Scope  NumInputPorts=9
  Scope{1..9} (9 alike) : Scope  NumInputPorts=2
  cmp_{1..9} (9 alike) : UnitTest_Lib/RoughlyEqual  slope=0.1
  result_tws : ToWorkspace  VariableName=spec_result_001
  tws_1 : ToWorkspace  VariableName=spec_req_001_001
  tws_2 : ToWorkspace  VariableName=spec_req_001_002
  tws_3 : ToWorkspace  VariableName=spec_req_001_003
  tws_4 : ToWorkspace  VariableName=spec_req_001_004
  tws_5 : ToWorkspace  VariableName=spec_req_001_005
  tws_6 : ToWorkspace  VariableName=spec_req_001_006
  tws_7 : ToWorkspace  VariableName=spec_req_001_007
  tws_8 : ToWorkspace  VariableName=spec_req_001_008
  tws_9 : ToWorkspace  VariableName=spec_req_001_009
  result : Outport
  wires:
  sig_Req_Bus/1 -> BS_Req/1
  sig_Result_Bus/1 -> BS_Result/1
  AndN/1 -> result/1, result_tws/1
  BS_Req/1 -> cmp_1/1, Scope1/1  "<testSig_AccPed_trqDesAct>"
  BS_Result/1 -> cmp_1/2, Scope1/2  "<AccPed_trqDesAct>"
  cmp_1/1 -> Bitwise_And1/1
  Bitwise_And1/1 -> tws_1/1, AndN/1, Scope/1
  BS_Req/2 -> cmp_2/1, Scope2/1  "<testSig_VehMot_stPrpAccPed>"
  BS_Result/2 -> cmp_2/2, Scope2/2  "<VehMot_stPrpAccPed>"
  cmp_2/1 -> Bitwise_And2/1
  Bitwise_And2/1 -> tws_2/1, AndN/2, Scope/2
  BS_Req/3 -> cmp_3/1, Scope3/1  "<testSig_AccPed_facCompAcs>"
  BS_Result/3 -> cmp_3/2, Scope3/2  "<AccPed_facCompAcs>"
  cmp_3/1 -> Bitwise_And3/1
  Bitwise_And3/1 -> tws_3/1, AndN/3, Scope/3
  BS_Req/4 -> cmp_4/1, Scope4/1  "<testSig_AccPed_trqComp>"
  BS_Result/4 -> cmp_4/2, Scope4/2  "<AccPed_trqComp>"
  cmp_4/1 -> Bitwise_And4/1
  Bitwise_And4/1 -> tws_4/1, AndN/4, Scope/4
  BS_Req/5 -> cmp_5/1, Scope5/1  "<testSig_AccPed_stBrkDes>"
  BS_Result/5 -> cmp_5/2, Scope5/2  "<AccPed_stBrkDes>"
  cmp_5/1 -> Bitwise_And5/1
  Bitwise_And5/1 -> tws_5/1, AndN/5, Scope/5
  BS_Req/6 -> cmp_6/1, Scope6/1  "<testSig_AccPed_stBrkDes_mp>"
  BS_Result/6 -> cmp_6/2, Scope6/2  "<AccPed_stBrkDes_mp>"
  cmp_6/1 -> Bitwise_And6/1
  Bitwise_And6/1 -> tws_6/1, AndN/6, Scope/6
  BS_Req/7 -> cmp_7/1, Scope7/1  "<testSig_AccPed_trqDifBrk_mp>"
  BS_Result/7 -> cmp_7/2, Scope7/2  "<AccPed_trqDifBrk_mp>"
  cmp_7/1 -> Bitwise_And7/1
  Bitwise_And7/1 -> tws_7/1, AndN/7, Scope/7
  BS_Req/8 -> cmp_8/1, Scope8/1  "<testSig_AccPed_rBrk50_mp>"
  BS_Result/8 -> cmp_8/2, Scope8/2  "<AccPed_rBrk50_mp>"
  cmp_8/1 -> Bitwise_And8/1
  Bitwise_And8/1 -> tws_8/1, AndN/8, Scope/8
  BS_Req/9 -> cmp_9/1, Scope9/1  "<testSig_AccPed_trqDesPull>"
  BS_Result/9 -> cmp_9/2, Scope9/2  "<AccPed_trqDesPull>"
  cmp_9/1 -> Bitwise_And9/1
  Bitwise_And9/1 -> tws_9/1, AndN/9, Scope/9

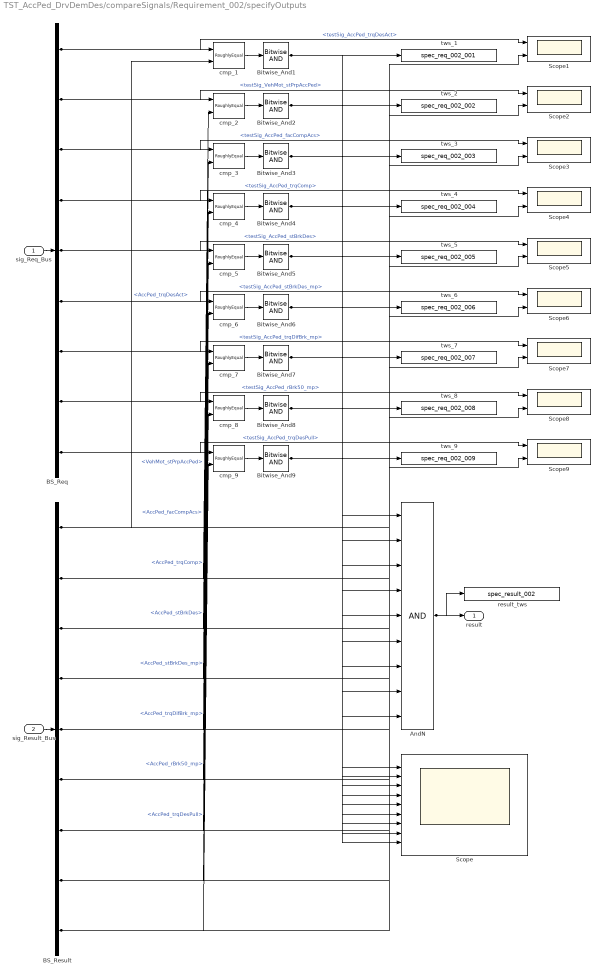
== system TST_AccPed_DrvDemDes/compareSignals/Requirement_002/specifyOutputs ==
  sig_Req_Bus : Inport
  sig_Result_Bus : Inport  Port=2
  AndN : Logic  Inputs=9
  BS_Req : BusSelector  OutputSignals=testSig_AccPed_trqDesAct,testSig_VehMot_stPrpAccPed,testSig_AccPed_facCompAcs,testSig_AccPed_trqComp,testSig_AccPed_stBrkDes,testSig_AccPed_stBrkDes_mp,testSig_AccPed_trqDifBrk_mp,testSig_AccPed_rBrk50_mp,testSig_AccPed_trqDesPull
  BS_Result : BusSelector  OutputSignals=AccPed_trqDesAct,VehMot_stPrpAccPed,AccPed_facCompAcs,AccPed_trqComp,AccPed_stBrkDes,AccPed_stBrkDes_mp,AccPed_trqDifBrk_mp,AccPed_rBrk50_mp,AccPed_trqDesPull
  Bitwise_And{1..9} (9 alike) : simulink/Logic and Bit Operations/Bitwise Operator  logicop=AND  UseBitMask=off  BitMask=bin2dec('11011001')  BitMaskRealWorld=Stored Integer
  Scope : Scope  NumInputPorts=9
  Scope{1..9} (9 alike) : Scope  NumInputPorts=2
  cmp_{1..9} (9 alike) : UnitTest_Lib/RoughlyEqual  slope=0.1
  result_tws : ToWorkspace  VariableName=spec_result_002
  tws_1 : ToWorkspace  VariableName=spec_req_002_001
  tws_2 : ToWorkspace  VariableName=spec_req_002_002
  tws_3 : ToWorkspace  VariableName=spec_req_002_003
  tws_4 : ToWorkspace  VariableName=spec_req_002_004
  tws_5 : ToWorkspace  VariableName=spec_req_002_005
  tws_6 : ToWorkspace  VariableName=spec_req_002_006
  tws_7 : ToWorkspace  VariableName=spec_req_002_007
  tws_8 : ToWorkspace  VariableName=spec_req_002_008
  tws_9 : ToWorkspace  VariableName=spec_req_002_009
  result : Outport
  wires:
  sig_Req_Bus/1 -> BS_Req/1
  sig_Result_Bus/1 -> BS_Result/1
  AndN/1 -> result/1, result_tws/1
  BS_Req/1 -> cmp_1/1, Scope1/1  "<testSig_AccPed_trqDesAct>"
  BS_Result/1 -> cmp_1/2, Scope1/2  "<AccPed_trqDesAct>"
  cmp_1/1 -> Bitwise_And1/1
  Bitwise_And1/1 -> tws_1/1, AndN/1, Scope/1
  BS_Req/2 -> cmp_2/1, Scope2/1  "<testSig_VehMot_stPrpAccPed>"
  BS_Result/2 -> cmp_2/2, Scope2/2  "<VehMot_stPrpAccPed>"
  cmp_2/1 -> Bitwise_And2/1
  Bitwise_And2/1 -> tws_2/1, AndN/2, Scope/2
  BS_Req/3 -> cmp_3/1, Scope3/1  "<testSig_AccPed_facCompAcs>"
  BS_Result/3 -> cmp_3/2, Scope3/2  "<AccPed_facCompAcs>"
  cmp_3/1 -> Bitwise_And3/1
  Bitwise_And3/1 -> tws_3/1, AndN/3, Scope/3
  BS_Req/4 -> cmp_4/1, Scope4/1  "<testSig_AccPed_trqComp>"
  BS_Result/4 -> cmp_4/2, Scope4/2  "<AccPed_trqComp>"
  cmp_4/1 -> Bitwise_And4/1
  Bitwise_And4/1 -> tws_4/1, AndN/4, Scope/4
  BS_Req/5 -> cmp_5/1, Scope5/1  "<testSig_AccPed_stBrkDes>"
  BS_Result/5 -> cmp_5/2, Scope5/2  "<AccPed_stBrkDes>"
  cmp_5/1 -> Bitwise_And5/1
  Bitwise_And5/1 -> tws_5/1, AndN/5, Scope/5
  BS_Req/6 -> cmp_6/1, Scope6/1  "<testSig_AccPed_stBrkDes_mp>"
  BS_Result/6 -> cmp_6/2, Scope6/2  "<AccPed_stBrkDes_mp>"
  cmp_6/1 -> Bitwise_And6/1
  Bitwise_And6/1 -> tws_6/1, AndN/6, Scope/6
  BS_Req/7 -> cmp_7/1, Scope7/1  "<testSig_AccPed_trqDifBrk_mp>"
  BS_Result/7 -> cmp_7/2, Scope7/2  "<AccPed_trqDifBrk_mp>"
  cmp_7/1 -> Bitwise_And7/1
  Bitwise_And7/1 -> tws_7/1, AndN/7, Scope/7
  BS_Req/8 -> cmp_8/1, Scope8/1  "<testSig_AccPed_rBrk50_mp>"
  BS_Result/8 -> cmp_8/2, Scope8/2  "<AccPed_rBrk50_mp>"
  cmp_8/1 -> Bitwise_And8/1
  Bitwise_And8/1 -> tws_8/1, AndN/8, Scope/8
  BS_Req/9 -> cmp_9/1, Scope9/1  "<testSig_AccPed_trqDesPull>"
  BS_Result/9 -> cmp_9/2, Scope9/2  "<AccPed_trqDesPull>"
  cmp_9/1 -> Bitwise_And9/1
  Bitwise_And9/1 -> tws_9/1, AndN/9, Scope/9

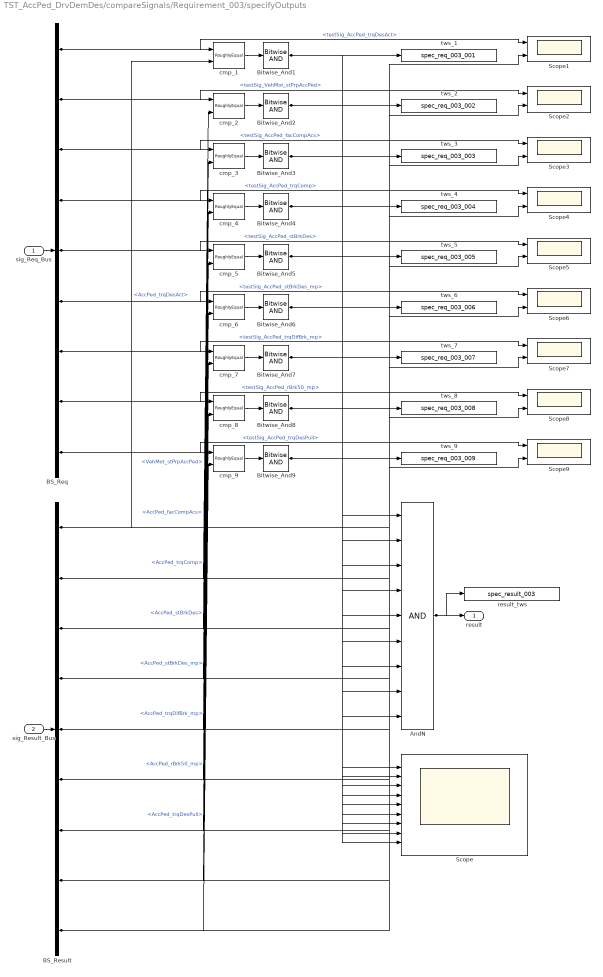
== system TST_AccPed_DrvDemDes/compareSignals/Requirement_003/specifyOutputs ==
  sig_Req_Bus : Inport
  sig_Result_Bus : Inport  Port=2
  AndN : Logic  Inputs=9
  BS_Req : BusSelector  OutputSignals=testSig_AccPed_trqDesAct,testSig_VehMot_stPrpAccPed,testSig_AccPed_facCompAcs,testSig_AccPed_trqComp,testSig_AccPed_stBrkDes,testSig_AccPed_stBrkDes_mp,testSig_AccPed_trqDifBrk_mp,testSig_AccPed_rBrk50_mp,testSig_AccPed_trqDesPull
  BS_Result : BusSelector  OutputSignals=AccPed_trqDesAct,VehMot_stPrpAccPed,AccPed_facCompAcs,AccPed_trqComp,AccPed_stBrkDes,AccPed_stBrkDes_mp,AccPed_trqDifBrk_mp,AccPed_rBrk50_mp,AccPed_trqDesPull
  Bitwise_And{1..9} (9 alike) : simulink/Logic and Bit Operations/Bitwise Operator  logicop=AND  UseBitMask=off  BitMask=bin2dec('11011001')  BitMaskRealWorld=Stored Integer
  Scope : Scope  NumInputPorts=9
  Scope{1..9} (9 alike) : Scope  NumInputPorts=2
  cmp_{1..9} (9 alike) : UnitTest_Lib/RoughlyEqual  slope=0.1
  result_tws : ToWorkspace  VariableName=spec_result_003
  tws_1 : ToWorkspace  VariableName=spec_req_003_001
  tws_2 : ToWorkspace  VariableName=spec_req_003_002
  tws_3 : ToWorkspace  VariableName=spec_req_003_003
  tws_4 : ToWorkspace  VariableName=spec_req_003_004
  tws_5 : ToWorkspace  VariableName=spec_req_003_005
  tws_6 : ToWorkspace  VariableName=spec_req_003_006
  tws_7 : ToWorkspace  VariableName=spec_req_003_007
  tws_8 : ToWorkspace  VariableName=spec_req_003_008
  tws_9 : ToWorkspace  VariableName=spec_req_003_009
  result : Outport
  wires:
  sig_Req_Bus/1 -> BS_Req/1
  sig_Result_Bus/1 -> BS_Result/1
  AndN/1 -> result/1, result_tws/1
  BS_Req/1 -> cmp_1/1, Scope1/1  "<testSig_AccPed_trqDesAct>"
  BS_Result/1 -> cmp_1/2, Scope1/2  "<AccPed_trqDesAct>"
  cmp_1/1 -> Bitwise_And1/1
  Bitwise_And1/1 -> tws_1/1, AndN/1, Scope/1
  BS_Req/2 -> cmp_2/1, Scope2/1  "<testSig_VehMot_stPrpAccPed>"
  BS_Result/2 -> cmp_2/2, Scope2/2  "<VehMot_stPrpAccPed>"
  cmp_2/1 -> Bitwise_And2/1
  Bitwise_And2/1 -> tws_2/1, AndN/2, Scope/2
  BS_Req/3 -> cmp_3/1, Scope3/1  "<testSig_AccPed_facCompAcs>"
  BS_Result/3 -> cmp_3/2, Scope3/2  "<AccPed_facCompAcs>"
  cmp_3/1 -> Bitwise_And3/1
  Bitwise_And3/1 -> tws_3/1, AndN/3, Scope/3
  BS_Req/4 -> cmp_4/1, Scope4/1  "<testSig_AccPed_trqComp>"
  BS_Result/4 -> cmp_4/2, Scope4/2  "<AccPed_trqComp>"
  cmp_4/1 -> Bitwise_And4/1
  Bitwise_And4/1 -> tws_4/1, AndN/4, Scope/4
  BS_Req/5 -> cmp_5/1, Scope5/1  "<testSig_AccPed_stBrkDes>"
  BS_Result/5 -> cmp_5/2, Scope5/2  "<AccPed_stBrkDes>"
  cmp_5/1 -> Bitwise_And5/1
  Bitwise_And5/1 -> tws_5/1, AndN/5, Scope/5
  BS_Req/6 -> cmp_6/1, Scope6/1  "<testSig_AccPed_stBrkDes_mp>"
  BS_Result/6 -> cmp_6/2, Scope6/2  "<AccPed_stBrkDes_mp>"
  cmp_6/1 -> Bitwise_And6/1
  Bitwise_And6/1 -> tws_6/1, AndN/6, Scope/6
  BS_Req/7 -> cmp_7/1, Scope7/1  "<testSig_AccPed_trqDifBrk_mp>"
  BS_Result/7 -> cmp_7/2, Scope7/2  "<AccPed_trqDifBrk_mp>"
  cmp_7/1 -> Bitwise_And7/1
  Bitwise_And7/1 -> tws_7/1, AndN/7, Scope/7
  BS_Req/8 -> cmp_8/1, Scope8/1  "<testSig_AccPed_rBrk50_mp>"
  BS_Result/8 -> cmp_8/2, Scope8/2  "<AccPed_rBrk50_mp>"
  cmp_8/1 -> Bitwise_And8/1
  Bitwise_And8/1 -> tws_8/1, AndN/8, Scope/8
  BS_Req/9 -> cmp_9/1, Scope9/1  "<testSig_AccPed_trqDesPull>"
  BS_Result/9 -> cmp_9/2, Scope9/2  "<AccPed_trqDesPull>"
  cmp_9/1 -> Bitwise_And9/1
  Bitwise_And9/1 -> tws_9/1, AndN/9, Scope/9

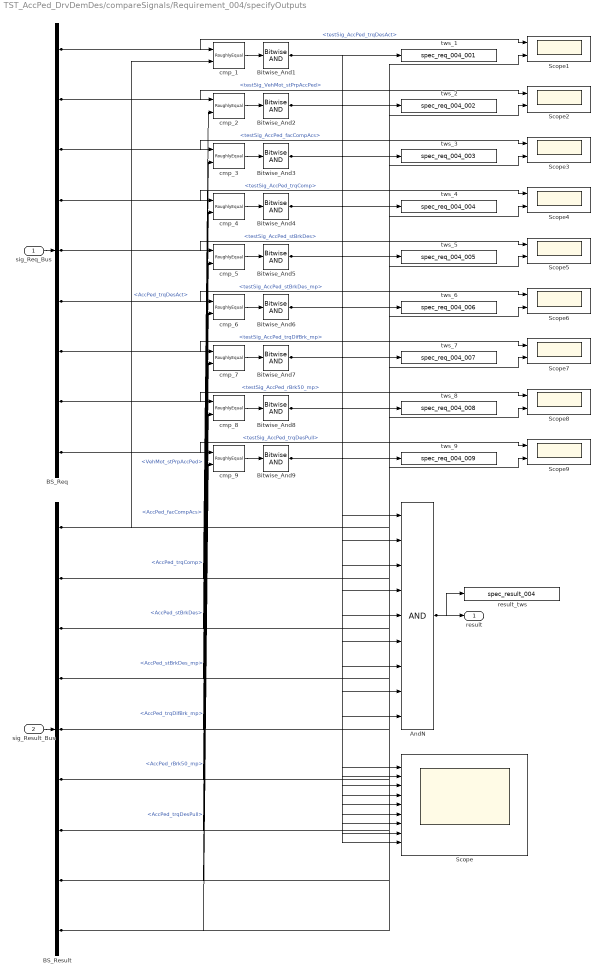
== system TST_AccPed_DrvDemDes/compareSignals/Requirement_004/specifyOutputs ==
  sig_Req_Bus : Inport
  sig_Result_Bus : Inport  Port=2
  AndN : Logic  Inputs=9
  BS_Req : BusSelector  OutputSignals=testSig_AccPed_trqDesAct,testSig_VehMot_stPrpAccPed,testSig_AccPed_facCompAcs,testSig_AccPed_trqComp,testSig_AccPed_stBrkDes,testSig_AccPed_stBrkDes_mp,testSig_AccPed_trqDifBrk_mp,testSig_AccPed_rBrk50_mp,testSig_AccPed_trqDesPull
  BS_Result : BusSelector  OutputSignals=AccPed_trqDesAct,VehMot_stPrpAccPed,AccPed_facCompAcs,AccPed_trqComp,AccPed_stBrkDes,AccPed_stBrkDes_mp,AccPed_trqDifBrk_mp,AccPed_rBrk50_mp,AccPed_trqDesPull
  Bitwise_And{1..9} (9 alike) : simulink/Logic and Bit Operations/Bitwise Operator  logicop=AND  UseBitMask=off  BitMask=bin2dec('11011001')  BitMaskRealWorld=Stored Integer
  Scope : Scope  NumInputPorts=9
  Scope{1..9} (9 alike) : Scope  NumInputPorts=2
  cmp_{1..9} (9 alike) : UnitTest_Lib/RoughlyEqual  slope=0.1
  result_tws : ToWorkspace  VariableName=spec_result_004
  tws_1 : ToWorkspace  VariableName=spec_req_004_001
  tws_2 : ToWorkspace  VariableName=spec_req_004_002
  tws_3 : ToWorkspace  VariableName=spec_req_004_003
  tws_4 : ToWorkspace  VariableName=spec_req_004_004
  tws_5 : ToWorkspace  VariableName=spec_req_004_005
  tws_6 : ToWorkspace  VariableName=spec_req_004_006
  tws_7 : ToWorkspace  VariableName=spec_req_004_007
  tws_8 : ToWorkspace  VariableName=spec_req_004_008
  tws_9 : ToWorkspace  VariableName=spec_req_004_009
  result : Outport
  wires:
  sig_Req_Bus/1 -> BS_Req/1
  sig_Result_Bus/1 -> BS_Result/1
  AndN/1 -> result/1, result_tws/1
  BS_Req/1 -> cmp_1/1, Scope1/1  "<testSig_AccPed_trqDesAct>"
  BS_Result/1 -> cmp_1/2, Scope1/2  "<AccPed_trqDesAct>"
  cmp_1/1 -> Bitwise_And1/1
  Bitwise_And1/1 -> tws_1/1, AndN/1, Scope/1
  BS_Req/2 -> cmp_2/1, Scope2/1  "<testSig_VehMot_stPrpAccPed>"
  BS_Result/2 -> cmp_2/2, Scope2/2  "<VehMot_stPrpAccPed>"
  cmp_2/1 -> Bitwise_And2/1
  Bitwise_And2/1 -> tws_2/1, AndN/2, Scope/2
  BS_Req/3 -> cmp_3/1, Scope3/1  "<testSig_AccPed_facCompAcs>"
  BS_Result/3 -> cmp_3/2, Scope3/2  "<AccPed_facCompAcs>"
  cmp_3/1 -> Bitwise_And3/1
  Bitwise_And3/1 -> tws_3/1, AndN/3, Scope/3
  BS_Req/4 -> cmp_4/1, Scope4/1  "<testSig_AccPed_trqComp>"
  BS_Result/4 -> cmp_4/2, Scope4/2  "<AccPed_trqComp>"
  cmp_4/1 -> Bitwise_And4/1
  Bitwise_And4/1 -> tws_4/1, AndN/4, Scope/4
  BS_Req/5 -> cmp_5/1, Scope5/1  "<testSig_AccPed_stBrkDes>"
  BS_Result/5 -> cmp_5/2, Scope5/2  "<AccPed_stBrkDes>"
  cmp_5/1 -> Bitwise_And5/1
  Bitwise_And5/1 -> tws_5/1, AndN/5, Scope/5
  BS_Req/6 -> cmp_6/1, Scope6/1  "<testSig_AccPed_stBrkDes_mp>"
  BS_Result/6 -> cmp_6/2, Scope6/2  "<AccPed_stBrkDes_mp>"
  cmp_6/1 -> Bitwise_And6/1
  Bitwise_And6/1 -> tws_6/1, AndN/6, Scope/6
  BS_Req/7 -> cmp_7/1, Scope7/1  "<testSig_AccPed_trqDifBrk_mp>"
  BS_Result/7 -> cmp_7/2, Scope7/2  "<AccPed_trqDifBrk_mp>"
  cmp_7/1 -> Bitwise_And7/1
  Bitwise_And7/1 -> tws_7/1, AndN/7, Scope/7
  BS_Req/8 -> cmp_8/1, Scope8/1  "<testSig_AccPed_rBrk50_mp>"
  BS_Result/8 -> cmp_8/2, Scope8/2  "<AccPed_rBrk50_mp>"
  cmp_8/1 -> Bitwise_And8/1
  Bitwise_And8/1 -> tws_8/1, AndN/8, Scope/8
  BS_Req/9 -> cmp_9/1, Scope9/1  "<testSig_AccPed_trqDesPull>"
  BS_Result/9 -> cmp_9/2, Scope9/2  "<AccPed_trqDesPull>"
  cmp_9/1 -> Bitwise_And9/1
  Bitwise_And9/1 -> tws_9/1, AndN/9, Scope/9

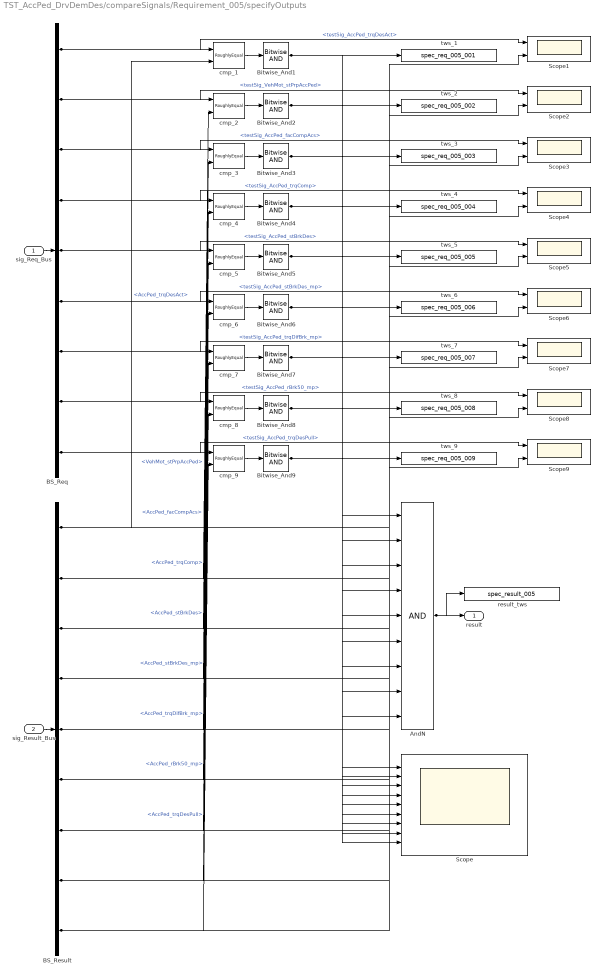
== system TST_AccPed_DrvDemDes/compareSignals/Requirement_005/specifyOutputs ==
  sig_Req_Bus : Inport
  sig_Result_Bus : Inport  Port=2
  AndN : Logic  Inputs=9
  BS_Req : BusSelector  OutputSignals=testSig_AccPed_trqDesAct,testSig_VehMot_stPrpAccPed,testSig_AccPed_facCompAcs,testSig_AccPed_trqComp,testSig_AccPed_stBrkDes,testSig_AccPed_stBrkDes_mp,testSig_AccPed_trqDifBrk_mp,testSig_AccPed_rBrk50_mp,testSig_AccPed_trqDesPull
  BS_Result : BusSelector  OutputSignals=AccPed_trqDesAct,VehMot_stPrpAccPed,AccPed_facCompAcs,AccPed_trqComp,AccPed_stBrkDes,AccPed_stBrkDes_mp,AccPed_trqDifBrk_mp,AccPed_rBrk50_mp,AccPed_trqDesPull
  Bitwise_And{1..9} (9 alike) : simulink/Logic and Bit Operations/Bitwise Operator  logicop=AND  UseBitMask=off  BitMask=bin2dec('11011001')  BitMaskRealWorld=Stored Integer
  Scope : Scope  NumInputPorts=9
  Scope{1..9} (9 alike) : Scope  NumInputPorts=2
  cmp_{1..9} (9 alike) : UnitTest_Lib/RoughlyEqual  slope=0.1
  result_tws : ToWorkspace  VariableName=spec_result_005
  tws_1 : ToWorkspace  VariableName=spec_req_005_001
  tws_2 : ToWorkspace  VariableName=spec_req_005_002
  tws_3 : ToWorkspace  VariableName=spec_req_005_003
  tws_4 : ToWorkspace  VariableName=spec_req_005_004
  tws_5 : ToWorkspace  VariableName=spec_req_005_005
  tws_6 : ToWorkspace  VariableName=spec_req_005_006
  tws_7 : ToWorkspace  VariableName=spec_req_005_007
  tws_8 : ToWorkspace  VariableName=spec_req_005_008
  tws_9 : ToWorkspace  VariableName=spec_req_005_009
  result : Outport
  wires:
  sig_Req_Bus/1 -> BS_Req/1
  sig_Result_Bus/1 -> BS_Result/1
  AndN/1 -> result/1, result_tws/1
  BS_Req/1 -> cmp_1/1, Scope1/1  "<testSig_AccPed_trqDesAct>"
  BS_Result/1 -> cmp_1/2, Scope1/2  "<AccPed_trqDesAct>"
  cmp_1/1 -> Bitwise_And1/1
  Bitwise_And1/1 -> tws_1/1, AndN/1, Scope/1
  BS_Req/2 -> cmp_2/1, Scope2/1  "<testSig_VehMot_stPrpAccPed>"
  BS_Result/2 -> cmp_2/2, Scope2/2  "<VehMot_stPrpAccPed>"
  cmp_2/1 -> Bitwise_And2/1
  Bitwise_And2/1 -> tws_2/1, AndN/2, Scope/2
  BS_Req/3 -> cmp_3/1, Scope3/1  "<testSig_AccPed_facCompAcs>"
  BS_Result/3 -> cmp_3/2, Scope3/2  "<AccPed_facCompAcs>"
  cmp_3/1 -> Bitwise_And3/1
  Bitwise_And3/1 -> tws_3/1, AndN/3, Scope/3
  BS_Req/4 -> cmp_4/1, Scope4/1  "<testSig_AccPed_trqComp>"
  BS_Result/4 -> cmp_4/2, Scope4/2  "<AccPed_trqComp>"
  cmp_4/1 -> Bitwise_And4/1
  Bitwise_And4/1 -> tws_4/1, AndN/4, Scope/4
  BS_Req/5 -> cmp_5/1, Scope5/1  "<testSig_AccPed_stBrkDes>"
  BS_Result/5 -> cmp_5/2, Scope5/2  "<AccPed_stBrkDes>"
  cmp_5/1 -> Bitwise_And5/1
  Bitwise_And5/1 -> tws_5/1, AndN/5, Scope/5
  BS_Req/6 -> cmp_6/1, Scope6/1  "<testSig_AccPed_stBrkDes_mp>"
  BS_Result/6 -> cmp_6/2, Scope6/2  "<AccPed_stBrkDes_mp>"
  cmp_6/1 -> Bitwise_And6/1
  Bitwise_And6/1 -> tws_6/1, AndN/6, Scope/6
  BS_Req/7 -> cmp_7/1, Scope7/1  "<testSig_AccPed_trqDifBrk_mp>"
  BS_Result/7 -> cmp_7/2, Scope7/2  "<AccPed_trqDifBrk_mp>"
  cmp_7/1 -> Bitwise_And7/1
  Bitwise_And7/1 -> tws_7/1, AndN/7, Scope/7
  BS_Req/8 -> cmp_8/1, Scope8/1  "<testSig_AccPed_rBrk50_mp>"
  BS_Result/8 -> cmp_8/2, Scope8/2  "<AccPed_rBrk50_mp>"
  cmp_8/1 -> Bitwise_And8/1
  Bitwise_And8/1 -> tws_8/1, AndN/8, Scope/8
  BS_Req/9 -> cmp_9/1, Scope9/1  "<testSig_AccPed_trqDesPull>"
  BS_Result/9 -> cmp_9/2, Scope9/2  "<AccPed_trqDesPull>"
  cmp_9/1 -> Bitwise_And9/1
  Bitwise_And9/1 -> tws_9/1, AndN/9, Scope/9

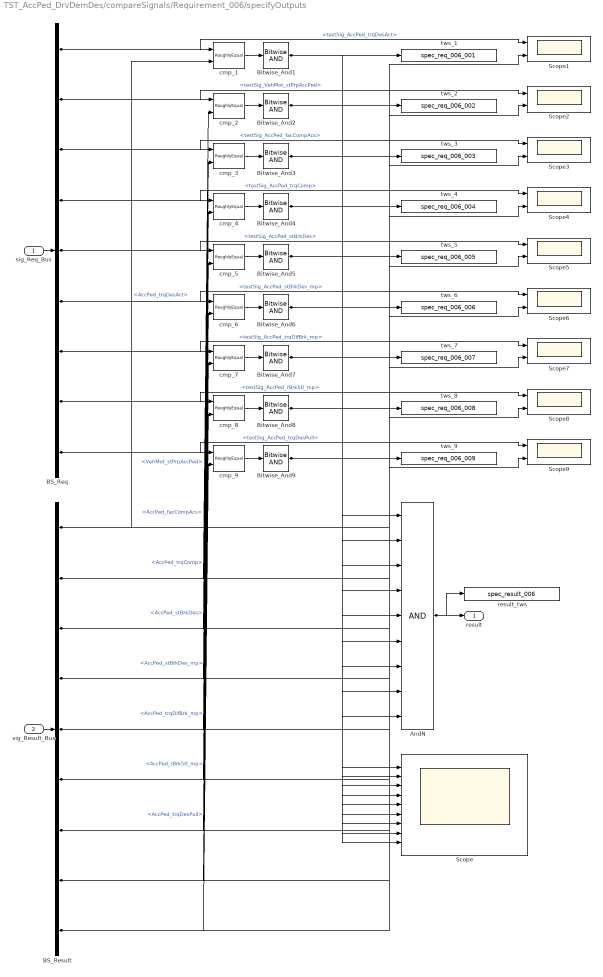
== system TST_AccPed_DrvDemDes/compareSignals/Requirement_006/specifyOutputs ==
  sig_Req_Bus : Inport
  sig_Result_Bus : Inport  Port=2
  AndN : Logic  Inputs=9
  BS_Req : BusSelector  OutputSignals=testSig_AccPed_trqDesAct,testSig_VehMot_stPrpAccPed,testSig_AccPed_facCompAcs,testSig_AccPed_trqComp,testSig_AccPed_stBrkDes,testSig_AccPed_stBrkDes_mp,testSig_AccPed_trqDifBrk_mp,testSig_AccPed_rBrk50_mp,testSig_AccPed_trqDesPull
  BS_Result : BusSelector  OutputSignals=AccPed_trqDesAct,VehMot_stPrpAccPed,AccPed_facCompAcs,AccPed_trqComp,AccPed_stBrkDes,AccPed_stBrkDes_mp,AccPed_trqDifBrk_mp,AccPed_rBrk50_mp,AccPed_trqDesPull
  Bitwise_And{1..9} (9 alike) : simulink/Logic and Bit Operations/Bitwise Operator  logicop=AND  UseBitMask=off  BitMask=bin2dec('11011001')  BitMaskRealWorld=Stored Integer
  Scope : Scope  NumInputPorts=9
  Scope{1..9} (9 alike) : Scope  NumInputPorts=2
  cmp_{1..9} (9 alike) : UnitTest_Lib/RoughlyEqual  slope=0.1
  result_tws : ToWorkspace  VariableName=spec_result_006
  tws_1 : ToWorkspace  VariableName=spec_req_006_001
  tws_2 : ToWorkspace  VariableName=spec_req_006_002
  tws_3 : ToWorkspace  VariableName=spec_req_006_003
  tws_4 : ToWorkspace  VariableName=spec_req_006_004
  tws_5 : ToWorkspace  VariableName=spec_req_006_005
  tws_6 : ToWorkspace  VariableName=spec_req_006_006
  tws_7 : ToWorkspace  VariableName=spec_req_006_007
  tws_8 : ToWorkspace  VariableName=spec_req_006_008
  tws_9 : ToWorkspace  VariableName=spec_req_006_009
  result : Outport
  wires:
  sig_Req_Bus/1 -> BS_Req/1
  sig_Result_Bus/1 -> BS_Result/1
  AndN/1 -> result/1, result_tws/1
  BS_Req/1 -> cmp_1/1, Scope1/1  "<testSig_AccPed_trqDesAct>"
  BS_Result/1 -> cmp_1/2, Scope1/2  "<AccPed_trqDesAct>"
  cmp_1/1 -> Bitwise_And1/1
  Bitwise_And1/1 -> tws_1/1, AndN/1, Scope/1
  BS_Req/2 -> cmp_2/1, Scope2/1  "<testSig_VehMot_stPrpAccPed>"
  BS_Result/2 -> cmp_2/2, Scope2/2  "<VehMot_stPrpAccPed>"
  cmp_2/1 -> Bitwise_And2/1
  Bitwise_And2/1 -> tws_2/1, AndN/2, Scope/2
  BS_Req/3 -> cmp_3/1, Scope3/1  "<testSig_AccPed_facCompAcs>"
  BS_Result/3 -> cmp_3/2, Scope3/2  "<AccPed_facCompAcs>"
  cmp_3/1 -> Bitwise_And3/1
  Bitwise_And3/1 -> tws_3/1, AndN/3, Scope/3
  BS_Req/4 -> cmp_4/1, Scope4/1  "<testSig_AccPed_trqComp>"
  BS_Result/4 -> cmp_4/2, Scope4/2  "<AccPed_trqComp>"
  cmp_4/1 -> Bitwise_And4/1
  Bitwise_And4/1 -> tws_4/1, AndN/4, Scope/4
  BS_Req/5 -> cmp_5/1, Scope5/1  "<testSig_AccPed_stBrkDes>"
  BS_Result/5 -> cmp_5/2, Scope5/2  "<AccPed_stBrkDes>"
  cmp_5/1 -> Bitwise_And5/1
  Bitwise_And5/1 -> tws_5/1, AndN/5, Scope/5
  BS_Req/6 -> cmp_6/1, Scope6/1  "<testSig_AccPed_stBrkDes_mp>"
  BS_Result/6 -> cmp_6/2, Scope6/2  "<AccPed_stBrkDes_mp>"
  cmp_6/1 -> Bitwise_And6/1
  Bitwise_And6/1 -> tws_6/1, AndN/6, Scope/6
  BS_Req/7 -> cmp_7/1, Scope7/1  "<testSig_AccPed_trqDifBrk_mp>"
  BS_Result/7 -> cmp_7/2, Scope7/2  "<AccPed_trqDifBrk_mp>"
  cmp_7/1 -> Bitwise_And7/1
  Bitwise_And7/1 -> tws_7/1, AndN/7, Scope/7
  BS_Req/8 -> cmp_8/1, Scope8/1  "<testSig_AccPed_rBrk50_mp>"
  BS_Result/8 -> cmp_8/2, Scope8/2  "<AccPed_rBrk50_mp>"
  cmp_8/1 -> Bitwise_And8/1
  Bitwise_And8/1 -> tws_8/1, AndN/8, Scope/8
  BS_Req/9 -> cmp_9/1, Scope9/1  "<testSig_AccPed_trqDesPull>"
  BS_Result/9 -> cmp_9/2, Scope9/2  "<AccPed_trqDesPull>"
  cmp_9/1 -> Bitwise_And9/1
  Bitwise_And9/1 -> tws_9/1, AndN/9, Scope/9
